simulink model "Path"  (R2024b)
settings: Solver=ode1  StartTime=0.0  StopTime=10.0  FixedStep=0.0005  RelTol=1e-3
values from neighbouring files (symbols this model uses):
  xi = 57.8    [Path_dd.sldd]
  xj = 56.5    [Path_dd.sldd]
  yi = 119.8    [Path_dd.sldd]
  yj = 118.0    [Path_dd.sldd]
  zi = 0.0    [Path_dd.sldd]
  zj = 0.0    [Path_dd.sldd]
settings Model: DataDictionary=Path_dd.sldd  EnableAccessToBaseWorkspace=off  Creator=wai484  LastModifiedBy=wai484
settings DataIOCC: SaveOutput=off  SaveTime=off
settings ModelReferenceCC: EnableParallelModelReferenceBuilds=on  ModelReferenceMinAlgLoopOccurrences=on
settings RTWCC: BuildConfiguration=Faster Runs
settings GRTTargetCC: CombineOutputUpdateFcns=off  OptimizeReductions=on

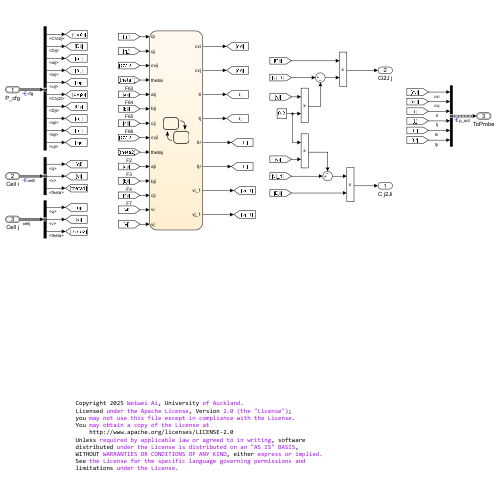
[thumbnail: Simulink's stored preview of the top-level diagram]
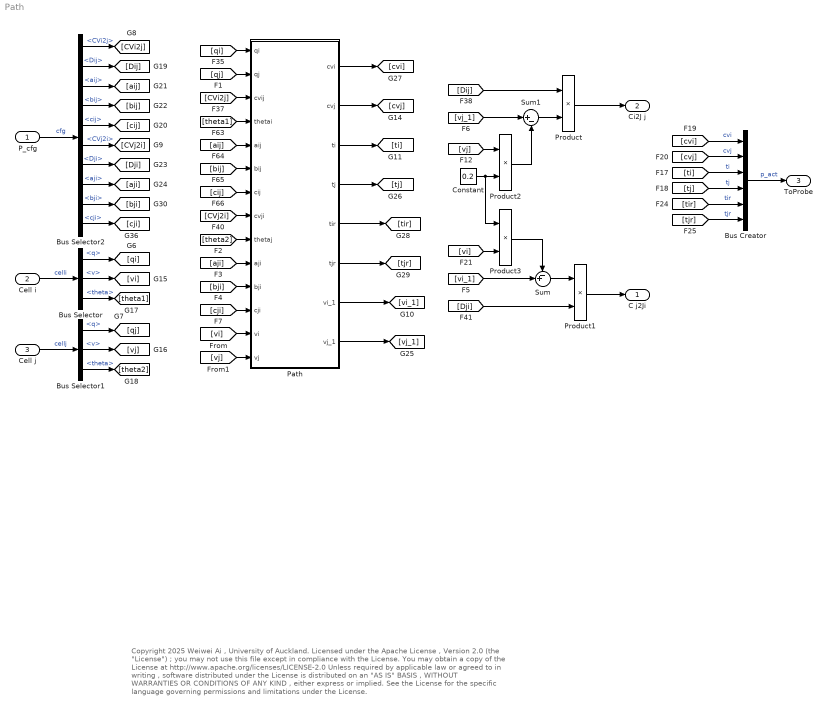
== system Path ==
  note: Copyright 2025 Weiwei Ai , University of Auckland.
      | Licensed under the Apache License , Version 2.0 (the "License") ;
      | you may not use this file except in compliance with the License.
      | You may obtain a copy of the License at
      | http://www.apache.org/licenses/LICENSE-2.0
      | Unless required by applicable law or agreed to in writing , software
      | distributed under the License is distributed on an "AS IS" BASIS ,
      | WITHOUT WARRANTIES OR CONDITIONS OF ANY KIND , either express or implied.
      | See the License for the specific language governing permissions and
      | limitations under the License.
  P_cfg : Inport  OutDataTypeStr=Bus: Config
  Cell i : Inport  Port=2  OutDataTypeStr=Bus: Cell
  Cell j : Inport  Port=3  OutDataTypeStr=Bus: Cell
  Bus Creator : BusCreator  Inputs=6  OutDataTypeStr=Bus: Activation  NonVirtualBus=on
      settings: InheritFromInputs=off
  Bus Selector : BusSelector  OutputSignals=q,v,theta
  Bus Selector1 : BusSelector  OutputSignals=q,v,theta
  Bus Selector2 : BusSelector  OutputSignals=CVi2j,Dij,aij,bij,cij,CVj2i,Dji,aji,bji,cji
  Constant : Constant  Value=0.2
  Path : Stateflow chart  TreatAsAtomicUnit=on
  Product{,1..3} (4 alike) : Product  Inputs=**
  Sum : Sum  Inputs=-+|
  Sum1 : Sum  Inputs=|+-
  C j2Ji : Outport  OutDataTypeStr=double  PortDimensions=1  SampleTime=[0.00050000000000000001,0]
  Ci2J j : Outport  Port=2  OutDataTypeStr=double  PortDimensions=1  SampleTime=[0.00050000000000000001,0]
  ToProbe : Outport  Port=3  OutDataTypeStr=Bus: Activation
  wires:
  Cell j/1 -> Bus Selector1/1  "cellj"
  Product/1 -> Ci2J j/1
  Product1/1 -> C j2Ji/1
  [qi] -> Path/1(qi)
  [Dij] -> Product/1
  [theta1] -> Path/4(thetai)
  [aij] -> Path/5(aij)
  [bij] -> Path/6(bij)
  [cij] -> Path/7(cij)
  [CVi2j] -> Path/3(cvij)
  [cji] -> Path/12(cji)
  [bji] -> Path/11(bji)
  [aji] -> Path/10(aji)
  [theta2] -> Path/9(thetaj)
  [CVj2i] -> Path/8(cvji)
  [qj] -> Path/2(qj)
  Path/8(vj_1) -> [vj_1]
  Path/7(vi_1) -> [vi_1]
  Path/1(cvi) -> [cvi]
  Path/2(cvj) -> [cvj]
  Path/3(ti) -> [ti]
  Path/4(tj) -> [tj]
  Path/5(tir) -> [tir]
  Path/6(tjr) -> [tjr]
  [vj_1] -> Sum1/1
  Sum1/1 -> Product/2
  [vj] -> Product2/1
  Product2/1 -> Sum1/2
  Constant/1 -> Product2/2, Product3/1
  Sum/1 -> Product1/1
  Product3/1 -> Sum/1
  [vi_1] -> Sum/2
  [Dji] -> Product1/2
  [vi] -> Product3/2
  Cell i/1 -> Bus Selector/1  "celli"
  Bus Selector/1 -> [qi]  "<q>"
  Bus Selector/2 -> [vi]  "<v>"
  Bus Selector/3 -> [theta1]  "<theta>"
  Bus Selector1/2 -> [vj]  "<v>"
  Bus Selector1/1 -> [qj]  "<q>"
  Bus Selector1/3 -> [theta2]  "<theta>"
  P_cfg/1 -> Bus Selector2/1  "cfg"
  Bus Selector2/1 -> [CVi2j]  "<CVi2j>"
  Bus Selector2/2 -> [Dij]  "<Dij>"
  Bus Selector2/3 -> [aij]  "<aij>"
  Bus Selector2/4 -> [bij]  "<bij>"
  Bus Selector2/5 -> [cij]  "<cij>"
  Bus Selector2/6 -> [CVj2i]  "<CVj2i>"
  Bus Selector2/7 -> [Dji]  "<Dji>"
  Bus Selector2/8 -> [aji]  "<aji>"
  Bus Selector2/9 -> [bji]  "<bji>"
  Bus Selector2/10 -> [cji]  "<cji>"
  [vi] -> Path/13(vi)
  [vj] -> Path/14(vj)
  Bus Creator/1 -> ToProbe/1  "p_act"
  [tir] -> Bus Creator/5  "tir"
  [tjr] -> Bus Creator/6  "tjr"
  [cvi] -> Bus Creator/1  "cvi"
  [cvj] -> Bus Creator/2  "cvj"
  [ti] -> Bus Creator/3  "ti"
  [tj] -> Bus Creator/4  "tj"

== stateflow chart Path/Path ==
  settings: updateMethod=DISCRETE
  state Wave
    state Relay_i [parallel]
      settings: executionOrder=8
      state Relay
        en: tj_1=0;
        du: tj_1=temporalCount(sec);
        vj_1=vbi(floor(tj_1)+1);
        ex: tj_1=0;
      state Idle
        en:
        vj_1=0;
      Wave.Relay_i.Idle -> Wave.Relay_i.Relay : Reach_j
      (default) -> Wave.Relay_i.Idle
      Wave.Relay_i.Relay -> Wave.Relay_i.Idle : [qj>=2 || j_1==0 ]
    state Cell_i [parallel]
      settings: executionOrder=5
      state Activation
      state Rest
        en:
        i_1=0;
      Wave.Cell_i.Rest -> Wave.Cell_i.Activation : Reach_i
      Wave.Cell_i.Activation -> Wave.Cell_i.Rest [order 1] : [after(tbj,sec)]
      (default) -> Wave.Cell_i.Rest
      Wave.Cell_i.Activation -> Wave.Cell_i.Rest [order 2] : Go_j
    state Relay_j [parallel]
      settings: executionOrder=7
      state Relay
        en: ti_1=0;
        du: ti_1=temporalCount(sec);
        vi_1=vbj(floor(ti_1)+1);
        ex: ti_1=0;
      state Idle
        en:
        vi_1=0;
      Wave.Relay_j.Idle -> Wave.Relay_j.Relay : Reach_i
      (default) -> Wave.Relay_j.Idle
      Wave.Relay_j.Relay -> Wave.Relay_j.Idle : [qi>=2 || i_1==0 ]
    state Cell_j [parallel]
      settings: executionOrder=6
      state Activation
      state Rest
        en:
        j_1=0;
      note: 1.
      Wave.Cell_j.Rest -> Wave.Cell_j.Activation : Reach_j
      Wave.Cell_j.Activation -> Wave.Cell_j.Rest [order 1] : [after(tbi,sec)]
      (default) -> Wave.Cell_j.Rest
      Wave.Cell_j.Activation -> Wave.Cell_j.Rest [order 2] : Go_i
    state End_j [parallel]
      settings: executionOrder=2
      state End_j_Idle
      state Go
        en: tj=0;
        du: tj=temporalCount(sec);
        ex: tj=0;
      note: 5
      state Ready
      note: 2.
      state BlockedByNeighbour
      Wave.End_j.Go -> Wave.End_j.End_j_Idle [order 2] : [Meet || mul==0]
      Wave.End_j.Go -> Wave.End_j.End_j_Idle [order 1] : [tj>=Tj && mul==1]
          | /{mul=mul-1;i_1=1; send(Reach_i,Cell_i);send(Reach_i,Relay_j);}
      (default) -> Wave.End_j.End_j_Idle
      Wave.End_j.End_j_Idle -> Wave.End_j.Ready [order 1] : [qj==2 && j_1==0]
      Wave.End_j.Ready -> Wave.End_j.Go [order 2] : [qj==3 && j_1==0]
          | /{ cvj=thetafcn(cvji,thetaj,aji,bji,cji);
          | Tj=l/cvj; mul=mul+1; send(Go_j,Buffer_j);send(Go_j,Cell_i);}
      Wave.End_j.End_j_Idle -> Wave.End_j.BlockedByNeighbour [order 2] : [qj==2 && j_1==1]
      Wave.End_j.Ready -> Wave.End_j.BlockedByNeighbour [order 1] : [cvji==0 || (qj==3 && j_1==1)]{tj=0;}
      Wave.End_j.BlockedByNeighbour -> Wave.End_j.End_j_Idle : [qj==0]
    state End_i [parallel]
      settings: executionOrder=1
      state End_i_Idle
      state Go
        en:ti=0;
        du: ti=temporalCount(sec);
        ex: ti=0;
      note: 4
      state Ready
      note: 2.
      note: 7
      state BlockedByNeighbour
      Wave.End_i.Go -> Wave.End_i.End_i_Idle [order 2] : [cvi*ti+cvj*tj>=l && mul==2]/
          | { mul=0; send(Meet,End_j);send(Meet,Buffer_i);send(Meet,Buffer_j);}
      Wave.End_i.Go -> Wave.End_i.End_i_Idle [order 1] : [ti>=Ti && mul==1]
          | /{mul=mul-1; j_1=1; send(Reach_j,Cell_j);send(Reach_j,Relay_i);}
      (default) -> Wave.End_i.End_i_Idle
      Wave.End_i.End_i_Idle -> Wave.End_i.Ready [order 1] : [qi==2 && i_1==0]
      Wave.End_i.Ready -> Wave.End_i.Go [order 2] : [qi==3 && i_1==0]
          | /{ cvi=thetafcn(cvij,thetai,aij,bij,cij);
          | Ti=l/cvi; mul=mul+1;send(Go_i,Buffer_i);send(Go_i,Cell_j); }
      Wave.End_i.End_i_Idle -> Wave.End_i.BlockedByNeighbour [order 2] : [qi==2 && i_1==1]
      Wave.End_i.Ready -> Wave.End_i.BlockedByNeighbour [order 1] : [cvij==0 || (qi==3 && i_1==1)]{ti=0;}
      Wave.End_i.BlockedByNeighbour -> Wave.End_i.End_i_Idle : [qi==0]
    state Buffer_i [parallel]
      settings: executionOrder=3
      state Idle
      note: 6
      state Buffer_i
        en: tbi=0;
        du: tbi=temporalCount(sec);
        vbi(floor(tbi)+1)=vi;
      (default) -> Wave.Buffer_i.Idle
      Wave.Buffer_i.Idle -> Wave.Buffer_i.Buffer_i : Go_i
      Wave.Buffer_i.Buffer_i -> Wave.Buffer_i.Idle [order 1] : [qi<3]
      Wave.Buffer_i.Buffer_i -> Wave.Buffer_i.Idle [order 2] : Meet
      Wave.Buffer_i.Buffer_i -> Wave.Buffer_i.Idle [order 3] : [tbi>=0.599]
    note: 3
    state Buffer_j [parallel]
      settings: executionOrder=4
      state Idle
      state Buffer_i
        en: tbj=0;
        du: tbj=temporalCount(sec);
        vbj(floor(tbj)+1)=vj;
      (default) -> Wave.Buffer_j.Idle
      Wave.Buffer_j.Idle -> Wave.Buffer_j.Buffer_i : Go_j
      Wave.Buffer_j.Buffer_i -> Wave.Buffer_j.Idle [order 1] : [qj<3]
      Wave.Buffer_j.Buffer_i -> Wave.Buffer_j.Idle [order 2] : Meet
      Wave.Buffer_j.Buffer_i -> Wave.Buffer_j.Idle [order 3] : [tbj>=0.599]
    state End_i_Fade [parallel]
      settings: executionOrder=10
      state End_i_Idle
      state End_i_re
        du: tir=temporalCount(sec);
      End_i_re -> Wave.End_i_Fade.End_i_Idle [order 1] : [cvi*tir+cvj*tjr>=l && tjr~=0]
          | /{send(Meet_r,End_j_Fade);tir=0;tjr=0;}
      End_i_re -> Wave.End_i_Fade.End_i_Idle [order 2] : [cvi*tir+cvj*tjr>=l&& tjr==0]/{tir=0;}
      (default) -> Wave.End_i_Fade.End_i_Idle
      Wave.End_i_Fade.End_i_Idle -> End_i_re : cell_i_r
    state End_j_Fade [parallel]
      settings: executionOrder=12
      state End_j_Idle
      state End_j_re
        du: tjr=temporalCount(sec);
      End_j_re -> Wave.End_j_Fade.End_j_Idle [order 1] : [cvi*tir+cvj*tjr>=l&& tir==0]/{tjr=0;}
      End_j_re -> Wave.End_j_Fade.End_j_Idle [order 2] : Meet_r
      (default) -> Wave.End_j_Fade.End_j_Idle
      Wave.End_j_Fade.End_j_Idle -> End_j_re : cell_j_r
    state Celll_j_Re [parallel]
      settings: executionOrder=9
      state Re
      state De
      Wave.Celll_j_Re.De -> Wave.Celll_j_Re.Re : [qj==0]/{send(cell_j_r,End_j_Fade);}
      Wave.Celll_j_Re.Re -> Wave.Celll_j_Re.De : [qj==3]
      (default) -> Wave.Celll_j_Re.Re
    state Celll_i_Re [parallel]
      settings: executionOrder=11
      state Re
      state De
      Wave.Celll_i_Re.De -> Wave.Celll_i_Re.Re : [qi==0]/{send(cell_i_r,End_i_Fade);}
      Wave.Celll_i_Re.Re -> Wave.Celll_i_Re.De : [qi==3]
      (default) -> Wave.Celll_i_Re.Re
    note: 1. The Cell_j_1 will be released if it has been resting or another AP from Cell_i starts travelling;.
    note: 2. Cell_i start to repolarize before the activation either reaches Cell_j or meets the activation from Cell_j, which happens when the APD is short or/and the path is long, e.g., premature depolarization.
        | In this case, the path would ignore all following activation before the premature activation reaches Cell_j or meets the activation from Cell_j.
  note: 3. Assume that the APD<=600 ms; If the APD>600, it would be truncated; Store the action potential of q3 until it goes back to repolarization or meets the other one.
      | 4. j_1=1; and Reach_j must occur at the same time to block Go_j immediately;
      | 5. mul==0 to make sure the transition to take in case Meet event is missed
      | 6. qi<3 instead of qi==0 to avoid where qi==0 is missed due to the stimulation timing and the simulation step;
      | 7. when cv=0, no propagation.
  (default) -> Wave : /{l=sqrt((xj-xi)^2+(yj-yi)^2+(zj-zi)^2);
      | cvi=cvij;
      | cvj=cvji;
      | Ti=1/cvi;
      | Tj=1/cvj;
      | ti=0;
      | tj=0;
      | ti_1=0;
      | tj_1=0;
      | i_1=0;
      | j_1=0;
      | vi_1=0;
      | vj_1=0;
      | tir=0;
      | tjr=0;
      | tbi=0;
      | tbj=0;
      | vbi=zeros(1,600);
      | vbj=zeros(1,600);
      | mul=0;
      | }
  data: cvin function_input double; thetain function_input double; ain function_input double; bin function_input double; cin function_input double; cvout function_output double; cvi output double; cvj output double; ti output double; qi input; qj input; ti_1 local double; tj_1 local double; cvij input; thetai input; aij input; bij input; cij input; cvji input; thetaj input; aji input; bji input; cji input; tj output; tir output; tjr output; i_1 local; j_1 local; vi_1 output; vj_1 output; l local double; tbi local; tbj local; vbi local; vbj local; vi input; vj input; Ti local double; Tj local double; mul local; xi parameter; xj parameter; yi parameter; yj parameter; zi parameter; zj parameter
  events: Reach_i local FUNCTION_CALL_EVENT; Reach_j local FUNCTION_CALL_EVENT; Go_i local FUNCTION_CALL_EVENT; Go_j local FUNCTION_CALL_EVENT; Meet local FUNCTION_CALL_EVENT; Meet_r local FUNCTION_CALL_EVENT; cell_i_r local FUNCTION_CALL_EVENT; cell_j_r local FUNCTION_CALL_EVENT
  function cvout = thetafcn(cvin,thetain,ain,bin,cin):
    | function cvout = thetafcn(cvin,thetain,ain,bin,cin)
    | %#codegen
    | %Rate dependent factor
    | ftheta=1/(ain*exp(bin*thetain)+(1-ain)*exp(-cin*thetain));
    | cvout=cvin*ftheta;
    | end
